simulink model "tp_three"  (R2018a)
settings: Solver=VariableStepAuto  StartTime=0.0  StopTime=1  RelTol=1e-3
libraries: powerlib x13, powerlib_meascontrol x2
settings Model: Creator=MSC COMPUTER  LastModifiedBy=MSC COMPUTER

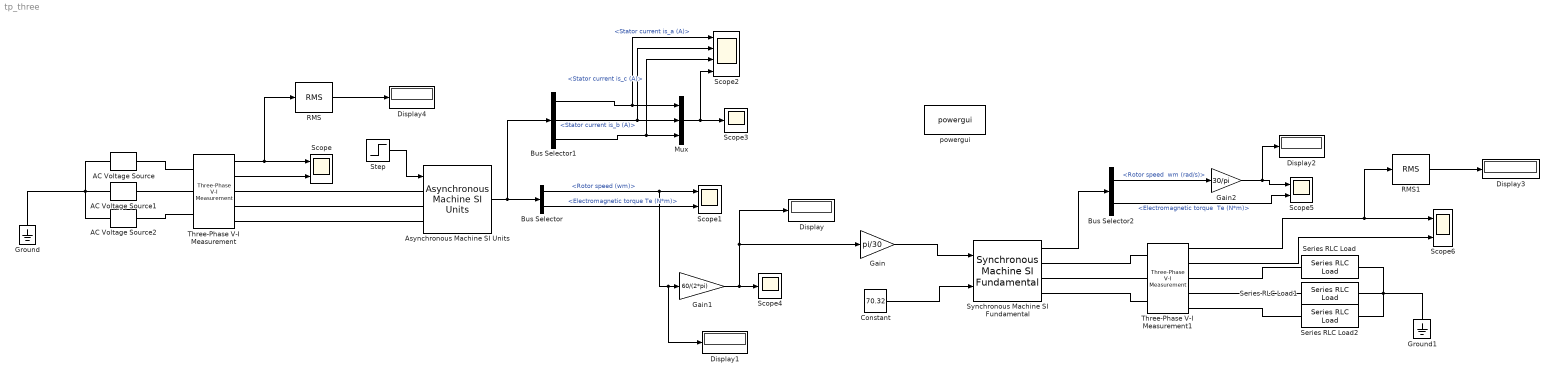
== system tp_three ==
  AC Voltage Source : powerlib/Electrical Sources/AC Voltage Source  Amplitude=240/(sqrt(3))*sqrt(2)  Phase=0  Frequency=6  SampleTime=0  Measurements=None  BusType=swing  Pref=10e3  Qref=0  Qmin=-inf  Qmax=+inf
  AC Voltage Source1 : powerlib/Electrical Sources/AC Voltage Source  Amplitude=240/(sqrt(3))*sqrt(2)  Phase=-120  Frequency=6  SampleTime=0  Measurements=None  BusType=swing  Pref=10e3  Qref=0  Qmin=-inf  Qmax=+inf
  AC Voltage Source2 : powerlib/Electrical Sources/AC Voltage Source  Amplitude=240/(sqrt(3))*sqrt(2)  Phase=120  Frequency=6  SampleTime=0  Measurements=None  BusType=swing  Pref=10e3  Qref=0  Qmin=-inf  Qmax=+inf
  Asynchronous Machine SI Units : powerlib/Machines/Asynchronous Machine SI Units  RotorType=Squirrel-cage  PresetModel=No  MechanicalLoad=Torque Tm  ShowDetailedParameters=on  ReferenceFrame=Rotor  Units=SI  MeasurementBus=off  NominalParameters=[1243.55 240 50]  Stator=[2.9 0.0125]  Rotor=[2.2 0.0125]  Cage1=[0.4155 0.002066]  Cage2=[0.4168 0.0003495]  Lm=0.29  Mechanical=[0.1 0 2]  PolePairs=2  InitialConditions=[1 0 0 0 0 0 120 2400]  SimulateSaturation=off  Saturation=[14.03593122, 27.81365428, 53.79336849, 72.68890987, 97.98006896, 148.6815601, 215.7428561, 302.9841135, 428.7778367 ; 230, 322, 414, 460, 506, 552, 598, 644, 690]  LoadFlowParameters=1492000  TsPowergui=0  TsBlock=-1  IterativeModel=Trapezoidal non iterative  IterativeDiscreteModel=Trapezoidal non iterative  Pmec=1.492e+006
  Bus Selector : BusSelector  OutputSignals=Mechanical.Rotor speed (wm),Mechanical.Electromagnetic torque Te (N*m)
  Bus Selector1 : BusSelector  OutputSignals=Stator measurements.Stator current is_a (A),Stator measurements.Stator current is_b (A),Stator measurements.Stator current is_c (A)
  Bus Selector2 : BusSelector  OutputSignals="Mechanical.Rotor speed  wm (rad/s),Mechanical.Electromagnetic torque  Te (N*m)"
  Constant : Constant  Value=70.32
  Display{,1..4} (5 alike) : Display
  Gain : Gain  Gain=pi/30
  Gain1 : Gain  Gain=60/(2*pi)
  Gain2 : Gain  Gain=30/pi
  Ground : powerlib/Elements/Ground  LConnTagsString=a
  Ground1 : powerlib/Elements/Ground  LConnTagsString=a
  Mux : Mux  Inputs=3
  RMS : powerlib_meascontrol/Measurements/RMS  TrueRMS=on  Freq=6  RMSInit=120  Ts=0
  RMS1 : powerlib_meascontrol/Measurements/RMS  TrueRMS=on  Freq=60  RMSInit=120  Ts=0
  Scope{,1,5..6} (4 alike) : Scope  NumInputPorts=2
  Scope2 : Scope  NumInputPorts=4
  Scope3 : Scope
  Scope4 : Scope
  Series RLC Load : powerlib/Elements/Series RLC Load  LConnTagsString=a  RConnTagsString=__new0  NominalVoltage=13800/sqrt(3)  NominalFrequency=60  ActivePower=1e4  InductivePower=0  CapacitivePower=0  Setx0=off  InitialVoltage=0  SetiL0=off  InitialCurrent=0  Measurements=None  LoadType=constant Z
  Series RLC Load1 : powerlib/Elements/Series RLC Load  LConnTagsString=a  RConnTagsString=__new0  NominalVoltage=13800/sqrt(3)  NominalFrequency=60  ActivePower=1e4  InductivePower=0  CapacitivePower=0  Setx0=off  InitialVoltage=0  SetiL0=off  InitialCurrent=0  Measurements=None  LoadType=constant Z
  Series RLC Load2 : powerlib/Elements/Series RLC Load  LConnTagsString=a  RConnTagsString=__new0  NominalVoltage=13800/sqrt(3)  NominalFrequency=60  ActivePower=1e4  InductivePower=0  CapacitivePower=0  Setx0=off  InitialVoltage=0  SetiL0=off  InitialCurrent=0  Measurements=None  LoadType=constant Z
  Step : Step  SampleTime=0
  Synchronous Machine SI Fundamental : powerlib/Machines/Synchronous Machine SI Fundamental  PresetModel=No  MechanicalLoad=Mechanical power Pm  ShowDetailedParameters=on  RotorType=Salient-pole  Units=SI fundamental parameters  MeasurementBus=off  NominalParameters="[ 187E6  13800   60   1087 ]"  Stator="[ 2.9069E-03  3.0892E-04  3.2164E-03  9.7153E-04 ]"  Field="[ 5.9013E-04  3.0712E-04 ]"  Dampers2=[ 0.0664, 1.387e-3, 0.0292, 6.896e-4, 7.907e-3, 2.477e-3]  Dampers1="[ 1.1900E-02  4.9076E-04  2.0081E-02  1.0365E-03 ]"  Mechanical=[ 3.895e6 0 20 ]  PolePairs=20  InitialConditions="[ 0  0  0  0  0  0  0  0  70.3192 ]"  SetSaturation=off  Saturation=[695.64,774.7,917.5,1001.6,1082.2,1175.9,1293.6,1430.2,1583.7;9660,10623,12243,13063,13757,14437,15180,15890,16567]  DisplayVfd=off  LoadFlowParameters=[1,0,0,0,0]  TsPowergui=0  TsBlock=-1  IterativeModel=Trapezoidal non iterative  IterativeDiscreteModel=Trapezoidal non iterative  BusType=PV  Pref=0  Qref=0  Qmin=-inf  Qmax=inf  PLF=0  QLF=0
      settings: SourceProductName=Simscape Power Systems  SourceProductBaseCode=PS
  Three-Phase V-I Measurement : powerlib/Measurements/Three-Phase V-I Measurement  VoltageMeasurement=phase-to-phase  SetLabelV=off  LabelV=Vabc  Vpu=off  VpuLL=off  CurrentMeasurement=yes  SetLabelI=off  LabelI=Iabc  Ipu=off  Pbase=100e6  Vbase=500e3  OutputType=Complex  PhasorSimulation=off  PSBequivalent=0
  Three-Phase V-I Measurement1 : powerlib/Measurements/Three-Phase V-I Measurement  VoltageMeasurement=phase-to-phase  SetLabelV=off  LabelV=Vabc  Vpu=off  VpuLL=off  CurrentMeasurement=yes  SetLabelI=off  LabelI=Iabc  Ipu=off  Pbase=100e6  Vbase=500e3  OutputType=Complex  PhasorSimulation=off  PSBequivalent=0
  powergui : powerlib/powergui  Priority=1  SimulationMode=Continuous  SampleTime=50e-6  frequency=60  Iterations=50  frequencyindice=60  Pbase=100e6  ErrMax=1e-4  UnitsV=kV  UnitsW=MW  buscounter=0  FunctionMessages=off  echomessages=off  EnableUseOfTLC=off  CurrentSourceSwitches=off  DisableSnubberDevices=off  DisableRonSwitches=off  DisableVfSwitches=off  DisplayEquations=off  SolverType=Tustin/Backward Euler (TBE)  Interpol=off  ExternalGateDelay=off  methode=off  Ts=100  x0status=blocks  SPID=on  SwTol=0  HookPort=off  RestoreLinks=warning  ResistiveCurrentMeasurement=off  Frange=[0:2:500]  Ylog=off  Xlog=on  ShowGrid=off  save=off  variable=ZData  structure=0  ZoomFFT=off  StartTime=0.0  cycles=1  DisplayStyle=1  fundamental=60  FreqAxis=off  MaxFrequency=1000  frequencyindicesteady=1  RmsSteady=1  display=off
  wires:
  Three-Phase V-I Measurement/1 -> RMS/1, Scope/1
  Three-Phase V-I Measurement/2 -> Scope/2
  Step/1 -> Asynchronous Machine SI Units/1
  Asynchronous Machine SI Units/1 -> Bus Selector1/1, Bus Selector/1
  Bus Selector/1 -> Display1/1, Gain1/1, Scope1/1  "<Rotor speed (wm)>"
  Bus Selector/2 -> Scope1/2  "<Electromagnetic torque Te (N*m)>"
  Bus Selector1/2 -> Scope2/2, Mux/2  "<Stator current is_b (A)>"
  Bus Selector1/3 -> Scope2/3, Mux/3  "<Stator current is_c (A)>"
  Bus Selector1/1 -> Scope2/1, Mux/1  "<Stator current is_a (A)>"
  Mux/1 -> Scope2/4, Scope3/1
  Gain/1 -> Synchronous Machine SI Fundamental/1
  Constant/1 -> Synchronous Machine SI Fundamental/2
  Gain1/1 -> Gain/1, Display/1, Scope4/1
  Synchronous Machine SI Fundamental/1 -> Bus Selector2/1
  Bus Selector2/1 -> Gain2/1  "<Rotor speed  wm (rad/s)>"
  Bus Selector2/2 -> Scope5/2  "<Electromagnetic torque  Te (N*m)>"
  Gain2/1 -> Display2/1, Scope5/1
  Three-Phase V-I Measurement1/1 -> RMS1/1, Scope6/1
  Three-Phase V-I Measurement1/2 -> Scope6/2
  RMS1/1 -> Display3/1
  RMS/1 -> Display4/1
  connections:
  AC Voltage Source2/RConn1 -- Three-Phase V-I Measurement/LConn3
  AC Voltage Source1/RConn1 -- Three-Phase V-I Measurement/LConn2
  AC Voltage Source/RConn1 -- Three-Phase V-I Measurement/LConn1
  Three-Phase V-I Measurement/RConn1 -- Asynchronous Machine SI Units/LConn1
  Three-Phase V-I Measurement/RConn2 -- Asynchronous Machine SI Units/LConn2
  Three-Phase V-I Measurement/RConn3 -- Asynchronous Machine SI Units/LConn3
  AC Voltage Source/LConn1 -- Ground/LConn1 -- AC Voltage Source1/LConn1 -- AC Voltage Source2/LConn1
  Synchronous Machine SI Fundamental/RConn2 -- Three-Phase V-I Measurement1/LConn2
  Synchronous Machine SI Fundamental/RConn1 -- Three-Phase V-I Measurement1/LConn1
  Synchronous Machine SI Fundamental/RConn3 -- Three-Phase V-I Measurement1/LConn3
  Three-Phase V-I Measurement1/RConn2 -- Series RLC Load1/LConn1
  Three-Phase V-I Measurement1/RConn1 -- Series RLC Load/LConn1
  Three-Phase V-I Measurement1/RConn3 -- Series RLC Load2/LConn1
  Series RLC Load/RConn1 -- Ground1/LConn1 -- Series RLC Load1/RConn1 -- Series RLC Load2/RConn1
